simulink model "VCU_CS75_12_27_test_log"  (R2014a)
settings: Solver=FixedStepDiscrete  StartTime=0.0  StopTime=25  FixedStep=0.0005  RelTol=1e-3
undefined symbols (not defined in the file or in its folder): ecucoder_acal, ErrorSumMax1, ErrorSumMax2, ErrorSumMax3, I1, I2, I3, I_SW01_L, LaterlAngleCommand, LDW, Log_ErrorSumMax1, Log_ErrorSumMax2, Log_I1, Log_I2, Log_P1, Log_P2, Log_Takeover, P1, P2, P3, RemoteAcc, RemoteAcclPosition
libraries: simulink x927, ec5744lib x40
(part 4 of 31)

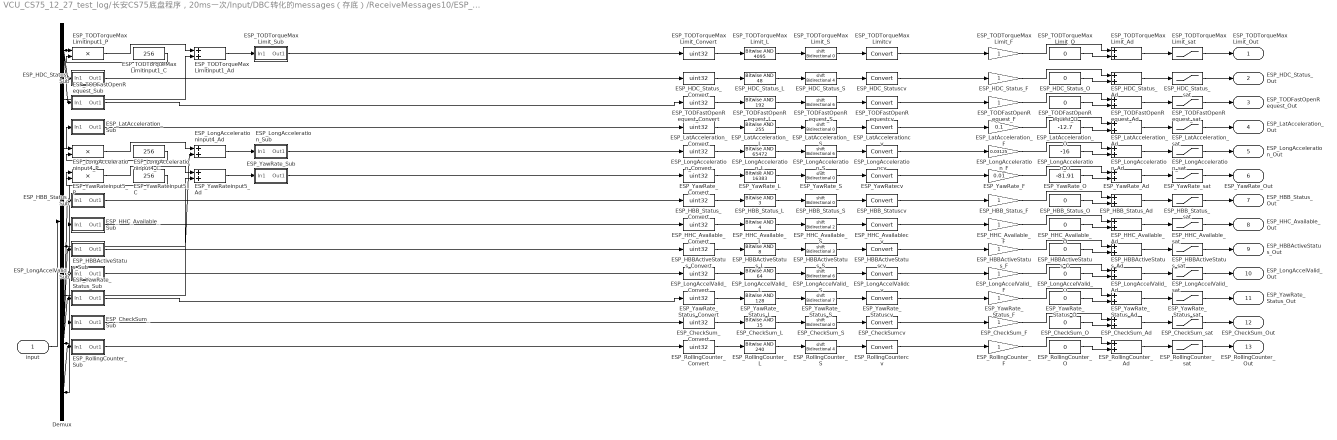
== system VCU_CS75_12_27_test_log/长安CS75底盘程序，20ms一次/Input/DBC转化的messages（存底）/ReceiveMessages10/ESP_287 ==
  input : Inport
  Demux : Demux  Outputs=8
  ESP_CheckSum_Ad : Sum
  ESP_CheckSum_Convert : DataTypeConversion  OutDataTypeStr=uint32
  ESP_CheckSum_F : Gain
  ESP_CheckSum_L : simulink/Logic and Bit Operations/Bitwise Operator  logicop=AND  UseBitMask=on  BitMask=15  BitMaskRealWorld=Stored Integer
  ESP_CheckSum_O : Constant  Value=0  OutDataTypeStr=single
  ESP_CheckSum_S : ArithShift
  ESP_CheckSum_Sub : Subsystem
  ESP_CheckSum_sat : Saturate  UpperLimit=15  LowerLimit=0
  ESP_CheckSumcv : DataTypeConversion
  ESP_HBBActiveStatus_Ad : Sum
  ESP_HBBActiveStatus_Convert : DataTypeConversion  OutDataTypeStr=uint32
  ESP_HBBActiveStatus_F : Gain
  ESP_HBBActiveStatus_L : simulink/Logic and Bit Operations/Bitwise Operator  logicop=AND  UseBitMask=on  BitMask=8  BitMaskRealWorld=Stored Integer
  ESP_HBBActiveStatus_O : Constant  Value=0  OutDataTypeStr=single
  ESP_HBBActiveStatus_S : ArithShift  BitShiftNumber=3
  ESP_HBBActiveStatus_Sub : Subsystem
  ESP_HBBActiveStatus_sat : Saturate  UpperLimit=1  LowerLimit=0
  ESP_HBBActiveStatuscv : DataTypeConversion
  ESP_HBB_Status_Ad : Sum
  ESP_HBB_Status_Convert : DataTypeConversion  OutDataTypeStr=uint32
  ESP_HBB_Status_F : Gain
  ESP_HBB_Status_L : simulink/Logic and Bit Operations/Bitwise Operator  logicop=AND  UseBitMask=on  BitMask=3  BitMaskRealWorld=Stored Integer
  ESP_HBB_Status_O : Constant  Value=0  OutDataTypeStr=single
  ESP_HBB_Status_S : ArithShift
  ESP_HBB_Status_Sub : Subsystem
  ESP_HBB_Status_sat : Saturate  UpperLimit=3  LowerLimit=0
  ESP_HBB_Statuscv : DataTypeConversion
  ESP_HDC_Status_Ad : Sum
  ESP_HDC_Status_Convert : DataTypeConversion  OutDataTypeStr=uint32
  ESP_HDC_Status_F : Gain
  ESP_HDC_Status_L : simulink/Logic and Bit Operations/Bitwise Operator  logicop=AND  UseBitMask=on  BitMask=48  BitMaskRealWorld=Stored Integer
  ESP_HDC_Status_O : Constant  Value=0  OutDataTypeStr=single
  ESP_HDC_Status_S : ArithShift  BitShiftNumber=4
  ESP_HDC_Status_Sub : Subsystem
  ESP_HDC_Status_sat : Saturate  UpperLimit=3  LowerLimit=0
  ESP_HDC_Statuscv : DataTypeConversion
  ESP_HHC_Available_Ad : Sum
  ESP_HHC_Available_Convert : DataTypeConversion  OutDataTypeStr=uint32
  ESP_HHC_Available_F : Gain
  ESP_HHC_Available_L : simulink/Logic and Bit Operations/Bitwise Operator  logicop=AND  UseBitMask=on  BitMask=4  BitMaskRealWorld=Stored Integer
  ESP_HHC_Available_O : Constant  Value=0  OutDataTypeStr=single
  ESP_HHC_Available_S : ArithShift  BitShiftNumber=2
  ESP_HHC_Available_Sub : Subsystem
  ESP_HHC_Available_sat : Saturate  UpperLimit=1  LowerLimit=0
  ESP_HHC_Availablecv : DataTypeConversion
  ESP_LatAcceleration_Ad : Sum
  ESP_LatAcceleration_Convert : DataTypeConversion  OutDataTypeStr=uint32
  ESP_LatAcceleration_F : Gain  Gain=0.1
  ESP_LatAcceleration_L : simulink/Logic and Bit Operations/Bitwise Operator  logicop=AND  UseBitMask=on  BitMask=255  BitMaskRealWorld=Stored Integer
  ESP_LatAcceleration_O : Constant  Value=-12.7  OutDataTypeStr=single
  ESP_LatAcceleration_S : ArithShift
  ESP_LatAcceleration_Sub : Subsystem
  ESP_LatAcceleration_sat : Saturate  UpperLimit=12.7  LowerLimit=-12.7
  ESP_LatAccelerationcv : DataTypeConversion
  ESP_LongAccelValid_Ad : Sum
  ESP_LongAccelValid_Convert : DataTypeConversion  OutDataTypeStr=uint32
  ESP_LongAccelValid_F : Gain
  ESP_LongAccelValid_L : simulink/Logic and Bit Operations/Bitwise Operator  logicop=AND  UseBitMask=on  BitMask=64  BitMaskRealWorld=Stored Integer
  ESP_LongAccelValid_O : Constant  Value=0  OutDataTypeStr=single
  ESP_LongAccelValid_S : ArithShift  BitShiftNumber=6
  ESP_LongAccelValid_Sub : Subsystem
  ESP_LongAccelValid_sat : Saturate  UpperLimit=1  LowerLimit=0
  ESP_LongAccelValidcv : DataTypeConversion
  ESP_LongAcceleration_Ad : Sum
  ESP_LongAcceleration_Convert : DataTypeConversion  OutDataTypeStr=uint32
  ESP_LongAcceleration_F : Gain  Gain=0.03125
  ESP_LongAcceleration_L : simulink/Logic and Bit Operations/Bitwise Operator  logicop=AND  UseBitMask=on  BitMask=65472  BitMaskRealWorld=Stored Integer
  ESP_LongAcceleration_O : Constant  Value=-16  OutDataTypeStr=single
  ESP_LongAcceleration_S : ArithShift  BitShiftNumber=6
  ESP_LongAcceleration_Sub : Subsystem
  ESP_LongAcceleration_sat : Saturate  UpperLimit=15.96875  LowerLimit=-16
  ESP_LongAccelerationcv : DataTypeConversion
  ESP_LongAccelerationinput4_Ad : Sum
  ESP_LongAccelerationinput4_C : Constant  Value=256
  ESP_LongAccelerationinput4_P : Product
  ESP_RollingCounter_Ad : Sum
  ESP_RollingCounter_Convert : DataTypeConversion  OutDataTypeStr=uint32
  ESP_RollingCounter_F : Gain
  ESP_RollingCounter_L : simulink/Logic and Bit Operations/Bitwise Operator  logicop=AND  UseBitMask=on  BitMask=240  BitMaskRealWorld=Stored Integer
  ESP_RollingCounter_O : Constant  Value=0  OutDataTypeStr=single
  ESP_RollingCounter_S : ArithShift  BitShiftNumber=4
  ESP_RollingCounter_Sub : Subsystem
  ESP_RollingCounter_sat : Saturate  UpperLimit=15  LowerLimit=0
  ESP_RollingCountercv : DataTypeConversion
  ESP_TODFastOpenRequest_Ad : Sum
  ESP_TODFastOpenRequest_Convert : DataTypeConversion  OutDataTypeStr=uint32
  ESP_TODFastOpenRequest_F : Gain
  ESP_TODFastOpenRequest_L : simulink/Logic and Bit Operations/Bitwise Operator  logicop=AND  UseBitMask=on  BitMask=192  BitMaskRealWorld=Stored Integer
  ESP_TODFastOpenRequest_O : Constant  Value=0  OutDataTypeStr=single
  ESP_TODFastOpenRequest_S : ArithShift  BitShiftNumber=6
  ESP_TODFastOpenRequest_Sub : Subsystem
  ESP_TODFastOpenRequest_sat : Saturate  UpperLimit=3  LowerLimit=0
  ESP_TODFastOpenRequestcv : DataTypeConversion
  ESP_TODTorqueMaxLimit_Ad : Sum
  ESP_TODTorqueMaxLimit_Convert : DataTypeConversion  OutDataTypeStr=uint32
  ESP_TODTorqueMaxLimit_F : Gain
  ESP_TODTorqueMaxLimit_L : simulink/Logic and Bit Operations/Bitwise Operator  logicop=AND  UseBitMask=on  BitMask=4095  BitMaskRealWorld=Stored Integer
  ESP_TODTorqueMaxLimit_O : Constant  Value=0  OutDataTypeStr=single
  ESP_TODTorqueMaxLimit_S : ArithShift
  ESP_TODTorqueMaxLimit_Sub : Subsystem
  ESP_TODTorqueMaxLimit_sat : Saturate  UpperLimit=4095  LowerLimit=0
  ESP_TODTorqueMaxLimitcv : DataTypeConversion
  ESP_TODTorqueMaxLimitinput1_Ad : Sum
  ESP_TODTorqueMaxLimitinput1_C : Constant  Value=256
  ESP_TODTorqueMaxLimitinput1_P : Product
  ESP_YawRate_Ad : Sum
  ESP_YawRate_Convert : DataTypeConversion  OutDataTypeStr=uint32
  ESP_YawRate_F : Gain  Gain=0.01
  ESP_YawRate_L : simulink/Logic and Bit Operations/Bitwise Operator  logicop=AND  UseBitMask=on  BitMask=16383  BitMaskRealWorld=Stored Integer
  ESP_YawRate_O : Constant  Value=-81.91  OutDataTypeStr=single
  ESP_YawRate_S : ArithShift
  ESP_YawRate_Status_Ad : Sum
  ESP_YawRate_Status_Convert : DataTypeConversion  OutDataTypeStr=uint32
  ESP_YawRate_Status_F : Gain
  ESP_YawRate_Status_L : simulink/Logic and Bit Operations/Bitwise Operator  logicop=AND  UseBitMask=on  BitMask=128  BitMaskRealWorld=Stored Integer
  ESP_YawRate_Status_O : Constant  Value=0  OutDataTypeStr=single
  ESP_YawRate_Status_S : ArithShift  BitShiftNumber=7
  ESP_YawRate_Status_Sub : Subsystem
  ESP_YawRate_Status_sat : Saturate  UpperLimit=1  LowerLimit=0
  ESP_YawRate_Statuscv : DataTypeConversion
  ESP_YawRate_Sub : Subsystem
  ESP_YawRate_sat : Saturate  UpperLimit=81.91  LowerLimit=-81.91
  ESP_YawRatecv : DataTypeConversion
  ESP_YawRateinput5_Ad : Sum
  ESP_YawRateinput5_C : Constant  Value=256
  ESP_YawRateinput5_P : Product
  ESP_TODTorqueMaxLimit_Out : Outport
  ESP_HDC_Status_Out : Outport  Port=2
  ESP_TODFastOpenRequest_Out : Outport  Port=3
  ESP_LatAcceleration_Out : Outport  Port=4
  ESP_LongAcceleration_Out : Outport  Port=5
  ESP_YawRate_Out : Outport  Port=6
  ESP_HBB_Status_Out : Outport  Port=7
  ESP_HHC_Available_Out : Outport  Port=8
  ESP_HBBActiveStatus_Out : Outport  Port=9
  ESP_LongAccelValid_Out : Outport  Port=10
  ESP_YawRate_Status_Out : Outport  Port=11
  ESP_CheckSum_Out : Outport  Port=12
  ESP_RollingCounter_Out : Outport  Port=13
  wires:
  input/1 -> Demux/1
  ESP_RollingCountercv/1 -> ESP_RollingCounter_F/1
  ESP_RollingCounter_S/1 -> ESP_RollingCountercv/1
  ESP_RollingCounter_L/1 -> ESP_RollingCounter_S/1
  ESP_RollingCounter_Convert/1 -> ESP_RollingCounter_L/1
  ESP_RollingCounter_Sub/1(Out1) -> ESP_RollingCounter_Convert/1
  ESP_RollingCounter_sat/1 -> ESP_RollingCounter_Out/1
  ESP_RollingCounter_Ad/1 -> ESP_RollingCounter_sat/1
  ESP_RollingCounter_O/1 -> ESP_RollingCounter_Ad/2
  ESP_RollingCounter_F/1 -> ESP_RollingCounter_Ad/1
  ESP_CheckSumcv/1 -> ESP_CheckSum_F/1
  ESP_CheckSum_S/1 -> ESP_CheckSumcv/1
  ESP_CheckSum_L/1 -> ESP_CheckSum_S/1
  ESP_CheckSum_Convert/1 -> ESP_CheckSum_L/1
  ESP_CheckSum_Sub/1(Out1) -> ESP_CheckSum_Convert/1
  Demux/8 -> ESP_RollingCounter_Sub/1(In1), ESP_CheckSum_Sub/1(In1)
  ESP_CheckSum_sat/1 -> ESP_CheckSum_Out/1
  ESP_CheckSum_Ad/1 -> ESP_CheckSum_sat/1
  ESP_CheckSum_O/1 -> ESP_CheckSum_Ad/2
  ESP_CheckSum_F/1 -> ESP_CheckSum_Ad/1
  ESP_YawRate_Statuscv/1 -> ESP_YawRate_Status_F/1
  ESP_YawRate_Status_S/1 -> ESP_YawRate_Statuscv/1
  ESP_YawRate_Status_L/1 -> ESP_YawRate_Status_S/1
  ESP_YawRate_Status_Convert/1 -> ESP_YawRate_Status_L/1
  ESP_YawRate_Status_Sub/1(Out1) -> ESP_YawRate_Status_Convert/1
  ESP_YawRate_Status_sat/1 -> ESP_YawRate_Status_Out/1
  ESP_YawRate_Status_Ad/1 -> ESP_YawRate_Status_sat/1
  ESP_YawRate_Status_O/1 -> ESP_YawRate_Status_Ad/2
  ESP_YawRate_Status_F/1 -> ESP_YawRate_Status_Ad/1
  ESP_LongAccelValidcv/1 -> ESP_LongAccelValid_F/1
  ESP_LongAccelValid_S/1 -> ESP_LongAccelValidcv/1
  ESP_LongAccelValid_L/1 -> ESP_LongAccelValid_S/1
  ESP_LongAccelValid_Convert/1 -> ESP_LongAccelValid_L/1
  ESP_LongAccelValid_Sub/1(Out1) -> ESP_LongAccelValid_Convert/1
  ESP_LongAccelValid_sat/1 -> ESP_LongAccelValid_Out/1
  ESP_LongAccelValid_Ad/1 -> ESP_LongAccelValid_sat/1
  ESP_LongAccelValid_O/1 -> ESP_LongAccelValid_Ad/2
  ESP_LongAccelValid_F/1 -> ESP_LongAccelValid_Ad/1
  ESP_HBBActiveStatuscv/1 -> ESP_HBBActiveStatus_F/1
  ESP_HBBActiveStatus_S/1 -> ESP_HBBActiveStatuscv/1
  ESP_HBBActiveStatus_L/1 -> ESP_HBBActiveStatus_S/1
  ESP_HBBActiveStatus_Convert/1 -> ESP_HBBActiveStatus_L/1
  ESP_HBBActiveStatus_Sub/1(Out1) -> ESP_HBBActiveStatus_Convert/1
  ESP_HBBActiveStatus_sat/1 -> ESP_HBBActiveStatus_Out/1
  ESP_HBBActiveStatus_Ad/1 -> ESP_HBBActiveStatus_sat/1
  ESP_HBBActiveStatus_O/1 -> ESP_HBBActiveStatus_Ad/2
  ESP_HBBActiveStatus_F/1 -> ESP_HBBActiveStatus_Ad/1
  ESP_HHC_Availablecv/1 -> ESP_HHC_Available_F/1
  ESP_HHC_Available_S/1 -> ESP_HHC_Availablecv/1
  ESP_HHC_Available_L/1 -> ESP_HHC_Available_S/1
  ESP_HHC_Available_Convert/1 -> ESP_HHC_Available_L/1
  ESP_HHC_Available_Sub/1(Out1) -> ESP_HHC_Available_Convert/1
  ESP_HHC_Available_sat/1 -> ESP_HHC_Available_Out/1
  ESP_HHC_Available_Ad/1 -> ESP_HHC_Available_sat/1
  ESP_HHC_Available_O/1 -> ESP_HHC_Available_Ad/2
  ESP_HHC_Available_F/1 -> ESP_HHC_Available_Ad/1
  ESP_HBB_Statuscv/1 -> ESP_HBB_Status_F/1
  ESP_HBB_Status_S/1 -> ESP_HBB_Statuscv/1
  ESP_HBB_Status_L/1 -> ESP_HBB_Status_S/1
  ESP_HBB_Status_Convert/1 -> ESP_HBB_Status_L/1
  ESP_HBB_Status_Sub/1(Out1) -> ESP_HBB_Status_Convert/1
  Demux/7 -> ESP_YawRate_Status_Sub/1(In1), ESP_LongAccelValid_Sub/1(In1), ESP_HBBActiveStatus_Sub/1(In1), ESP_HHC_Available_Sub/1(In1), ESP_HBB_Status_Sub/1(In1)
  ESP_HBB_Status_sat/1 -> ESP_HBB_Status_Out/1
  ESP_HBB_Status_Ad/1 -> ESP_HBB_Status_sat/1
  ESP_HBB_Status_O/1 -> ESP_HBB_Status_Ad/2
  ESP_HBB_Status_F/1 -> ESP_HBB_Status_Ad/1
  ESP_YawRatecv/1 -> ESP_YawRate_F/1
  ESP_YawRate_S/1 -> ESP_YawRatecv/1
  ESP_YawRate_L/1 -> ESP_YawRate_S/1
  ESP_YawRate_Convert/1 -> ESP_YawRate_L/1
  ESP_YawRate_Sub/1(Out1) -> ESP_YawRate_Convert/1
  ESP_YawRateinput5_Ad/1 -> ESP_YawRate_Sub/1(In1)
  Demux/6 -> ESP_YawRateinput5_Ad/2
  ESP_YawRateinput5_P/1 -> ESP_YawRateinput5_Ad/1
  ESP_YawRateinput5_C/1 -> ESP_YawRateinput5_P/2
  ESP_YawRate_sat/1 -> ESP_YawRate_Out/1
  ESP_YawRate_Ad/1 -> ESP_YawRate_sat/1
  ESP_YawRate_O/1 -> ESP_YawRate_Ad/2
  ESP_YawRate_F/1 -> ESP_YawRate_Ad/1
  ESP_LongAccelerationcv/1 -> ESP_LongAcceleration_F/1
  ESP_LongAcceleration_S/1 -> ESP_LongAccelerationcv/1
  ESP_LongAcceleration_L/1 -> ESP_LongAcceleration_S/1
  ESP_LongAcceleration_Convert/1 -> ESP_LongAcceleration_L/1
  ESP_LongAcceleration_Sub/1(Out1) -> ESP_LongAcceleration_Convert/1
  ESP_LongAccelerationinput4_Ad/1 -> ESP_LongAcceleration_Sub/1(In1)
  Demux/5 -> ESP_YawRateinput5_P/1, ESP_LongAccelerationinput4_Ad/2
  ESP_LongAccelerationinput4_P/1 -> ESP_LongAccelerationinput4_Ad/1
  ESP_LongAccelerationinput4_C/1 -> ESP_LongAccelerationinput4_P/2
  Demux/4 -> ESP_LongAccelerationinput4_P/1
  ESP_LongAcceleration_sat/1 -> ESP_LongAcceleration_Out/1
  ESP_LongAcceleration_Ad/1 -> ESP_LongAcceleration_sat/1
  ESP_LongAcceleration_O/1 -> ESP_LongAcceleration_Ad/2
  ESP_LongAcceleration_F/1 -> ESP_LongAcceleration_Ad/1
  ESP_LatAccelerationcv/1 -> ESP_LatAcceleration_F/1
  ESP_LatAcceleration_S/1 -> ESP_LatAccelerationcv/1
  ESP_LatAcceleration_L/1 -> ESP_LatAcceleration_S/1
  ESP_LatAcceleration_Convert/1 -> ESP_LatAcceleration_L/1
  ESP_LatAcceleration_Sub/1(Out1) -> ESP_LatAcceleration_Convert/1
  Demux/3 -> ESP_LatAcceleration_Sub/1(In1)
  ESP_LatAcceleration_sat/1 -> ESP_LatAcceleration_Out/1
  ESP_LatAcceleration_Ad/1 -> ESP_LatAcceleration_sat/1
  ESP_LatAcceleration_O/1 -> ESP_LatAcceleration_Ad/2
  ESP_LatAcceleration_F/1 -> ESP_LatAcceleration_Ad/1
  ESP_TODFastOpenRequestcv/1 -> ESP_TODFastOpenRequest_F/1
  ESP_TODFastOpenRequest_S/1 -> ESP_TODFastOpenRequestcv/1
  ESP_TODFastOpenRequest_L/1 -> ESP_TODFastOpenRequest_S/1
  ESP_TODFastOpenRequest_Convert/1 -> ESP_TODFastOpenRequest_L/1
  ESP_TODFastOpenRequest_Sub/1(Out1) -> ESP_TODFastOpenRequest_Convert/1
  ESP_TODFastOpenRequest_sat/1 -> ESP_TODFastOpenRequest_Out/1
  ESP_TODFastOpenRequest_Ad/1 -> ESP_TODFastOpenRequest_sat/1
  ESP_TODFastOpenRequest_O/1 -> ESP_TODFastOpenRequest_Ad/2
  ESP_TODFastOpenRequest_F/1 -> ESP_TODFastOpenRequest_Ad/1
  ESP_HDC_Statuscv/1 -> ESP_HDC_Status_F/1
  ESP_HDC_Status_S/1 -> ESP_HDC_Statuscv/1
  ESP_HDC_Status_L/1 -> ESP_HDC_Status_S/1
  ESP_HDC_Status_Convert/1 -> ESP_HDC_Status_L/1
  ESP_HDC_Status_Sub/1(Out1) -> ESP_HDC_Status_Convert/1
  ESP_HDC_Status_sat/1 -> ESP_HDC_Status_Out/1
  ESP_HDC_Status_Ad/1 -> ESP_HDC_Status_sat/1
  ESP_HDC_Status_O/1 -> ESP_HDC_Status_Ad/2
  ESP_HDC_Status_F/1 -> ESP_HDC_Status_Ad/1
  ESP_TODTorqueMaxLimitcv/1 -> ESP_TODTorqueMaxLimit_F/1
  ESP_TODTorqueMaxLimit_S/1 -> ESP_TODTorqueMaxLimitcv/1
  ESP_TODTorqueMaxLimit_L/1 -> ESP_TODTorqueMaxLimit_S/1
  ESP_TODTorqueMaxLimit_Convert/1 -> ESP_TODTorqueMaxLimit_L/1
  ESP_TODTorqueMaxLimit_Sub/1(Out1) -> ESP_TODTorqueMaxLimit_Convert/1
  ESP_TODTorqueMaxLimitinput1_Ad/1 -> ESP_TODTorqueMaxLimit_Sub/1(In1)
  Demux/2 -> ESP_TODTorqueMaxLimitinput1_Ad/2
  ESP_TODTorqueMaxLimitinput1_P/1 -> ESP_TODTorqueMaxLimitinput1_Ad/1
  ESP_TODTorqueMaxLimitinput1_C/1 -> ESP_TODTorqueMaxLimitinput1_P/2
  Demux/1 -> ESP_TODFastOpenRequest_Sub/1(In1), ESP_HDC_Status_Sub/1(In1), ESP_TODTorqueMaxLimitinput1_P/1
  ESP_TODTorqueMaxLimit_sat/1 -> ESP_TODTorqueMaxLimit_Out/1
  ESP_TODTorqueMaxLimit_Ad/1 -> ESP_TODTorqueMaxLimit_sat/1
  ESP_TODTorqueMaxLimit_O/1 -> ESP_TODTorqueMaxLimit_Ad/2
  ESP_TODTorqueMaxLimit_F/1 -> ESP_TODTorqueMaxLimit_Ad/1

== system VCU_CS75_12_27_test_log/长安CS75底盘程序，20ms一次/Input/DBC转化的messages（存底）/ReceiveMessages11/HU_AEBSetting_551 ==
  input : Inport
  Demux : Demux  Outputs=8
  HU_AEBOnOffSetting_Ad : Sum
  HU_AEBOnOffSetting_Convert : DataTypeConversion  OutDataTypeStr=uint32
  HU_AEBOnOffSetting_F : Gain
  HU_AEBOnOffSetting_L : simulink/Logic and Bit Operations/Bitwise Operator  logicop=AND  UseBitMask=on  BitMask=8  BitMaskRealWorld=Stored Integer
  HU_AEBOnOffSetting_O : Constant  Value=0  OutDataTypeStr=single
  HU_AEBOnOffSetting_S : ArithShift  BitShiftNumber=3
  HU_AEBOnOffSetting_Sub : Subsystem
  HU_AEBOnOffSetting_sat : Saturate  UpperLimit=1  LowerLimit=0
  HU_AEBOnOffSettingcv : DataTypeConversion
  HU_FCWSetting_Ad : Sum
  HU_FCWSetting_Convert : DataTypeConversion  OutDataTypeStr=uint32
  HU_FCWSetting_F : Gain
  HU_FCWSetting_L : simulink/Logic and Bit Operations/Bitwise Operator  logicop=AND  UseBitMask=on  BitMask=24  BitMaskRealWorld=Stored Integer
  HU_FCWSetting_O : Constant  Value=0  OutDataTypeStr=single
  HU_FCWSetting_S : ArithShift  BitShiftNumber=3
  HU_FCWSetting_Sub : Subsystem
  HU_FCWSetting_sat : Saturate  UpperLimit=0  LowerLimit=0
  HU_FCWSettingcv : DataTypeConversion
  HU_LCASetting_Ad : Sum
  HU_LCASetting_Convert : DataTypeConversion  OutDataTypeStr=uint32
  HU_LCASetting_F : Gain
  HU_LCASetting_L : simulink/Logic and Bit Operations/Bitwise Operator  logicop=AND  UseBitMask=on  BitMask=3  BitMaskRealWorld=Stored Integer
  HU_LCASetting_O : Constant  Value=0  OutDataTypeStr=single
  HU_LCASetting_S : ArithShift
  HU_LCASetting_Sub : Subsystem
  HU_LCASetting_sat : Saturate  UpperLimit=0  LowerLimit=0
  HU_LCASettingcv : DataTypeConversion
  HU_AEBOnOffSetting_Out : Outport
  HU_LCASetting_Out : Outport  Port=2
  HU_FCWSetting_Out : Outport  Port=3
  wires:
  input/1 -> Demux/1
  HU_FCWSettingcv/1 -> HU_FCWSetting_F/1
  HU_FCWSetting_S/1 -> HU_FCWSettingcv/1
  HU_FCWSetting_L/1 -> HU_FCWSetting_S/1
  HU_FCWSetting_Convert/1 -> HU_FCWSetting_L/1
  HU_FCWSetting_Sub/1(Out1) -> HU_FCWSetting_Convert/1
  HU_FCWSetting_sat/1 -> HU_FCWSetting_Out/1
  HU_FCWSetting_Ad/1 -> HU_FCWSetting_sat/1
  HU_FCWSetting_O/1 -> HU_FCWSetting_Ad/2
  HU_FCWSetting_F/1 -> HU_FCWSetting_Ad/1
  HU_LCASettingcv/1 -> HU_LCASetting_F/1
  HU_LCASetting_S/1 -> HU_LCASettingcv/1
  HU_LCASetting_L/1 -> HU_LCASetting_S/1
  HU_LCASetting_Convert/1 -> HU_LCASetting_L/1
  HU_LCASetting_Sub/1(Out1) -> HU_LCASetting_Convert/1
  Demux/5 -> HU_FCWSetting_Sub/1(In1), HU_LCASetting_Sub/1(In1)
  HU_LCASetting_sat/1 -> HU_LCASetting_Out/1
  HU_LCASetting_Ad/1 -> HU_LCASetting_sat/1
  HU_LCASetting_O/1 -> HU_LCASetting_Ad/2
  HU_LCASetting_F/1 -> HU_LCASetting_Ad/1
  HU_AEBOnOffSettingcv/1 -> HU_AEBOnOffSetting_F/1
  HU_AEBOnOffSetting_S/1 -> HU_AEBOnOffSettingcv/1
  HU_AEBOnOffSetting_L/1 -> HU_AEBOnOffSetting_S/1
  HU_AEBOnOffSetting_Convert/1 -> HU_AEBOnOffSetting_L/1
  HU_AEBOnOffSetting_Sub/1(Out1) -> HU_AEBOnOffSetting_Convert/1
  Demux/1 -> HU_AEBOnOffSetting_Sub/1(In1)
  HU_AEBOnOffSetting_sat/1 -> HU_AEBOnOffSetting_Out/1
  HU_AEBOnOffSetting_Ad/1 -> HU_AEBOnOffSetting_sat/1
  HU_AEBOnOffSetting_O/1 -> HU_AEBOnOffSetting_Ad/2
  HU_AEBOnOffSetting_F/1 -> HU_AEBOnOffSetting_Ad/1

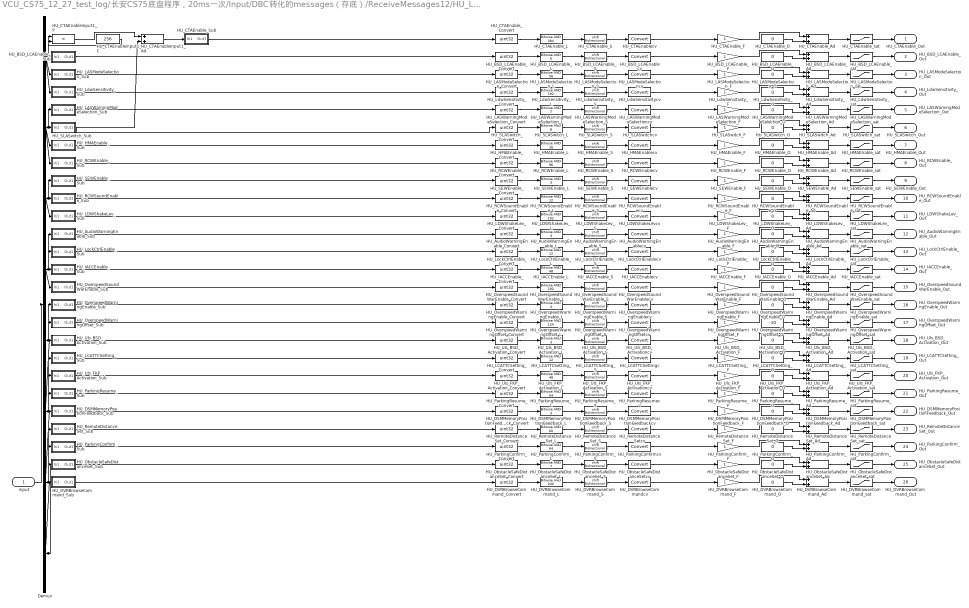
== system VCU_CS75_12_27_test_log/长安CS75底盘程序，20ms一次/Input/DBC转化的messages（存底）/ReceiveMessages12/HU_LASSetting_0x541 ==
  input : Inport
  Demux : Demux  Outputs=8
  HU_AudioWarningEnable_Ad : Sum
  HU_AudioWarningEnable_Convert : DataTypeConversion  OutDataTypeStr=uint32
  HU_AudioWarningEnable_F : Gain
  HU_AudioWarningEnable_L : simulink/Logic and Bit Operations/Bitwise Operator  logicop=AND  UseBitMask=on  BitMask=3  BitMaskRealWorld=Stored Integer
  HU_AudioWarningEnable_O : Constant  Value=0  OutDataTypeStr=single
  HU_AudioWarningEnable_S : ArithShift
  HU_AudioWarningEnable_Sub : Subsystem
  HU_AudioWarningEnable_sat : Saturate  UpperLimit=3  LowerLimit=0
  HU_AudioWarningEnablecv : DataTypeConversion
  HU_BSD_LCAEnable_Ad : Sum
  HU_BSD_LCAEnable_Convert : DataTypeConversion  OutDataTypeStr=uint32
  HU_BSD_LCAEnable_F : Gain
  HU_BSD_LCAEnable_L : simulink/Logic and Bit Operations/Bitwise Operator  logicop=AND  UseBitMask=on  BitMask=6  BitMaskRealWorld=Stored Integer
  HU_BSD_LCAEnable_O : Constant  Value=0  OutDataTypeStr=single
  HU_BSD_LCAEnable_S : ArithShift  BitShiftNumber=1
  HU_BSD_LCAEnable_Sub : Subsystem
  HU_BSD_LCAEnable_sat : Saturate  UpperLimit=3  LowerLimit=0
  HU_BSD_LCAEnablecv : DataTypeConversion
  HU_CTAEnable_Ad : Sum
  HU_CTAEnable_Convert : DataTypeConversion  OutDataTypeStr=uint32
  HU_CTAEnable_F : Gain
  HU_CTAEnable_L : simulink/Logic and Bit Operations/Bitwise Operator  logicop=AND  UseBitMask=on  BitMask=384  BitMaskRealWorld=Stored Integer
  HU_CTAEnable_O : Constant  Value=0  OutDataTypeStr=single
  HU_CTAEnable_S : ArithShift  BitShiftNumber=7
  HU_CTAEnable_Sub : Subsystem
  HU_CTAEnable_sat : Saturate  UpperLimit=3  LowerLimit=0
  HU_CTAEnablecv : DataTypeConversion
  HU_CTAEnableinput1_Ad : Sum
  HU_CTAEnableinput1_C : Constant  Value=256
  HU_CTAEnableinput1_P : Product
  HU_DSMMemoryPositionFeedback_Ad : Sum
  HU_DSMMemoryPositionFeedback_Convert : DataTypeConversion  OutDataTypeStr=uint32
  HU_DSMMemoryPositionFeedback_F : Gain
  HU_DSMMemoryPositionFeedback_L : simulink/Logic and Bit Operations/Bitwise Operator  logicop=AND  UseBitMask=on  BitMask=3  BitMaskRealWorld=Stored Integer
  HU_DSMMemoryPositionFeedback_O : Constant  Value=0  OutDataTypeStr=single
  HU_DSMMemoryPositionFeedback_S : ArithShift
  HU_DSMMemoryPositionFeedback_Sub : Subsystem
  HU_DSMMemoryPositionFeedback_sat : Saturate  UpperLimit=3  LowerLimit=0
  HU_DSMMemoryPositionFeedbackcv : DataTypeConversion
  HU_DVRBrowseCommand_Ad : Sum
  HU_DVRBrowseCommand_Convert : DataTypeConversion  OutDataTypeStr=uint32
  HU_DVRBrowseCommand_F : Gain
  HU_DVRBrowseCommand_L : simulink/Logic and Bit Operations/Bitwise Operator  logicop=AND  UseBitMask=on  BitMask=240  BitMaskRealWorld=Stored Integer
  HU_DVRBrowseCommand_O : Constant  Value=0  OutDataTypeStr=single
  HU_DVRBrowseCommand_S : ArithShift  BitShiftNumber=4
  HU_DVRBrowseCommand_Sub : Subsystem
  HU_DVRBrowseCommand_sat : Saturate  UpperLimit=15  LowerLimit=0
  HU_DVRBrowseCommandcv : DataTypeConversion
  HU_HMAEnable_Ad : Sum
  HU_HMAEnable_Convert : DataTypeConversion  OutDataTypeStr=uint32
  HU_HMAEnable_F : Gain
  HU_HMAEnable_L : simulink/Logic and Bit Operations/Bitwise Operator  logicop=AND  UseBitMask=on  BitMask=16  BitMaskRealWorld=Stored Integer
  HU_HMAEnable_O : Constant  Value=0  OutDataTypeStr=single
  HU_HMAEnable_S : ArithShift  BitShiftNumber=4
  HU_HMAEnable_Sub : Subsystem
  HU_HMAEnable_sat : Saturate  UpperLimit=1  LowerLimit=0
  HU_HMAEnablecv : DataTypeConversion
  HU_IACCEnable_Ad : Sum
  HU_IACCEnable_Convert : DataTypeConversion  OutDataTypeStr=uint32
  HU_IACCEnable_F : Gain
  HU_IACCEnable_L : simulink/Logic and Bit Operations/Bitwise Operator  logicop=AND  UseBitMask=on  BitMask=48  BitMaskRealWorld=Stored Integer
  HU_IACCEnable_O : Constant  Value=0  OutDataTypeStr=single
  HU_IACCEnable_S : ArithShift  BitShiftNumber=4
  HU_IACCEnable_Sub : Subsystem
  HU_IACCEnable_sat : Saturate  UpperLimit=3  LowerLimit=0
  HU_IACCEnablecv : DataTypeConversion
  HU_LASModeSelection_Ad : Sum
  HU_LASModeSelection_Convert : DataTypeConversion  OutDataTypeStr=uint32
  HU_LASModeSelection_F : Gain
  HU_LASModeSelection_L : simulink/Logic and Bit Operations/Bitwise Operator  logicop=AND  UseBitMask=on  BitMask=56  BitMaskRealWorld=Stored Integer
  HU_LASModeSelection_O : Constant  Value=0  OutDataTypeStr=single
  HU_LASModeSelection_S : ArithShift  BitShiftNumber=3
  HU_LASModeSelection_Sub : Subsystem
  HU_LASModeSelection_sat : Saturate  UpperLimit=7  LowerLimit=0
  HU_LASModeSelectioncv : DataTypeConversion
  HU_LASWarningModeSelection_Ad : Sum
  HU_LASWarningModeSelection_Convert : DataTypeConversion  OutDataTypeStr=uint32
  HU_LASWarningModeSelection_F : Gain
  HU_LASWarningModeSelection_L : simulink/Logic and Bit Operations/Bitwise Operator  logicop=AND  UseBitMask=on  BitMask=7  BitMaskRealWorld=Stored Integer
  HU_LASWarningModeSelection_O : Constant  Value=0  OutDataTypeStr=single
  HU_LASWarningModeSelection_S : ArithShift
  HU_LASWarningModeSelection_Sub : Subsystem
  HU_LASWarningModeSelection_sat : Saturate  UpperLimit=7  LowerLimit=0
  HU_LASWarningModeSelectioncv : DataTypeConversion
  HU_LCATTCSetting_Ad : Sum
  HU_LCATTCSetting_Convert : DataTypeConversion  OutDataTypeStr=uint32
  HU_LCATTCSetting_F : Gain
  HU_LCATTCSetting_L : simulink/Logic and Bit Operations/Bitwise Operator  logicop=AND  UseBitMask=on  BitMask=12  BitMaskRealWorld=Stored Integer
  HU_LCATTCSetting_O : Constant  Value=0  OutDataTypeStr=single
  HU_LCATTCSetting_S : ArithShift  BitShiftNumber=2
  HU_LCATTCSetting_Sub : Subsystem
  HU_LCATTCSetting_sat : Saturate  UpperLimit=3  LowerLimit=0
  HU_LCATTCSettingcv : DataTypeConversion
  HU_LDWShakeLev_Ad : Sum
  HU_LDWShakeLev_Convert : DataTypeConversion  OutDataTypeStr=uint32
  HU_LDWShakeLev_F : Gain
  HU_LDWShakeLev_L : simulink/Logic and Bit Operations/Bitwise Operator  logicop=AND  UseBitMask=on  BitMask=192  BitMaskRealWorld=Stored Integer
  HU_LDWShakeLev_O : Constant  Value=0  OutDataTypeStr=single
  HU_LDWShakeLev_S : ArithShift  BitShiftNumber=6
  HU_LDWShakeLev_Sub : Subsystem
  HU_LDWShakeLev_sat : Saturate  UpperLimit=3  LowerLimit=0
  HU_LDWShakeLevcv : DataTypeConversion
  HU_LdwSensitivity_Ad : Sum
  HU_LdwSensitivity_Convert : DataTypeConversion  OutDataTypeStr=uint32
  HU_LdwSensitivity_F : Gain
  HU_LdwSensitivity_L : simulink/Logic and Bit Operations/Bitwise Operator  logicop=AND  UseBitMask=on  BitMask=192  BitMaskRealWorld=Stored Integer
  HU_LdwSensitivity_O : Constant  Value=0  OutDataTypeStr=single
  HU_LdwSensitivity_S : ArithShift  BitShiftNumber=6
  HU_LdwSensitivity_Sub : Subsystem
  HU_LdwSensitivity_sat : Saturate  UpperLimit=3  LowerLimit=0
  HU_LdwSensitivitycv : DataTypeConversion
  HU_LockCtrlEnable_Ad : Sum
  HU_LockCtrlEnable_Convert : DataTypeConversion  OutDataTypeStr=uint32
  HU_LockCtrlEnable_F : Gain
  HU_LockCtrlEnable_L : simulink/Logic and Bit Operations/Bitwise Operator  logicop=AND  UseBitMask=on  BitMask=12  BitMaskRealWorld=Stored Integer
  HU_LockCtrlEnable_O : Constant  Value=0  OutDataTypeStr=single
  HU_LockCtrlEnable_S : ArithShift  BitShiftNumber=2
  HU_LockCtrlEnable_Sub : Subsystem
  HU_LockCtrlEnable_sat : Saturate  UpperLimit=3  LowerLimit=0
  HU_LockCtrlEnablecv : DataTypeConversion
  HU_ObstacleSafeDistanceSet_Ad : Sum
  HU_ObstacleSafeDistanceSet_Convert : DataTypeConversion  OutDataTypeStr=uint32
  HU_ObstacleSafeDistanceSet_F : Gain
  HU_ObstacleSafeDistanceSet_L : simulink/Logic and Bit Operations/Bitwise Operator  logicop=AND  UseBitMask=on  BitMask=7  BitMaskRealWorld=Stored Integer
  HU_ObstacleSafeDistanceSet_O : Constant  Value=0  OutDataTypeStr=single
  HU_ObstacleSafeDistanceSet_S : ArithShift
  HU_ObstacleSafeDistanceSet_Sub : Subsystem
  HU_ObstacleSafeDistanceSet_sat : Saturate  UpperLimit=7  LowerLimit=0
  HU_ObstacleSafeDistanceSetcv : DataTypeConversion
  HU_OverspeedSoundWarEnable_Ad : Sum
  HU_OverspeedSoundWarEnable_Convert : DataTypeConversion  OutDataTypeStr=uint32
  HU_OverspeedSoundWarEnable_F : Gain
  HU_OverspeedSoundWarEnable_L : simulink/Logic and Bit Operations/Bitwise Operator  logicop=AND  UseBitMask=on  BitMask=192  BitMaskRealWorld=Stored Integer
  HU_OverspeedSoundWarEnable_O : Constant  Value=0  OutDataTypeStr=single
  HU_OverspeedSoundWarEnable_S : ArithShift  BitShiftNumber=6
  HU_OverspeedSoundWarEnable_Sub : Subsystem
  HU_OverspeedSoundWarEnable_sat : Saturate  UpperLimit=3  LowerLimit=0
  HU_OverspeedSoundWarEnablecv : DataTypeConversion
  HU_OverspeedWarningEnable_Ad : Sum
  HU_OverspeedWarningEnable_Convert : DataTypeConversion  OutDataTypeStr=uint32
  HU_OverspeedWarningEnable_F : Gain
  HU_OverspeedWarningEnable_L : simulink/Logic and Bit Operations/Bitwise Operator  logicop=AND  UseBitMask=on  BitMask=3  BitMaskRealWorld=Stored Integer
  HU_OverspeedWarningEnable_O : Constant  Value=0  OutDataTypeStr=single
  HU_OverspeedWarningEnable_S : ArithShift
  HU_OverspeedWarningEnable_Sub : Subsystem
  HU_OverspeedWarningEnable_sat : Saturate  UpperLimit=3  LowerLimit=0
  HU_OverspeedWarningEnablecv : DataTypeConversion
  HU_OverspeedWarningOffset_Ad : Sum
  HU_OverspeedWarningOffset_Convert : DataTypeConversion  OutDataTypeStr=uint32
  HU_OverspeedWarningOffset_F : Gain
  HU_OverspeedWarningOffset_L : simulink/Logic and Bit Operations/Bitwise Operator  logicop=AND  UseBitMask=on  BitMask=124  BitMaskRealWorld=Stored Integer
  HU_OverspeedWarningOffset_O : Constant  Value=-10  OutDataTypeStr=single
  HU_OverspeedWarningOffset_S : ArithShift  BitShiftNumber=2
  HU_OverspeedWarningOffset_Sub : Subsystem
  HU_OverspeedWarningOffset_sat : Saturate  UpperLimit=10  LowerLimit=-10
  HU_OverspeedWarningOffsetcv : DataTypeConversion
  HU_ParkingConfirm_Ad : Sum
  HU_ParkingConfirm_Convert : DataTypeConversion  OutDataTypeStr=uint32
  HU_ParkingConfirm_F : Gain
  HU_ParkingConfirm_L : simulink/Logic and Bit Operations/Bitwise Operator  logicop=AND  UseBitMask=on  BitMask=64  BitMaskRealWorld=Stored Integer
  HU_ParkingConfirm_O : Constant  Value=0  OutDataTypeStr=single
  HU_ParkingConfirm_S : ArithShift  BitShiftNumber=6
  HU_ParkingConfirm_Sub : Subsystem
  HU_ParkingConfirm_sat : Saturate  UpperLimit=1  LowerLimit=0
  HU_ParkingConfirmcv : DataTypeConversion
  HU_ParkingResume_Ad : Sum
  HU_ParkingResume_Convert : DataTypeConversion  OutDataTypeStr=uint32
  HU_ParkingResume_F : Gain
  HU_ParkingResume_L : simulink/Logic and Bit Operations/Bitwise Operator  logicop=AND  UseBitMask=on  BitMask=64  BitMaskRealWorld=Stored Integer
  HU_ParkingResume_O : Constant  Value=0  OutDataTypeStr=single
  HU_ParkingResume_S : ArithShift  BitShiftNumber=6
  HU_ParkingResume_Sub : Subsystem
  HU_ParkingResume_sat : Saturate  UpperLimit=1  LowerLimit=0
  HU_ParkingResumecv : DataTypeConversion
  HU_RCWEnable_Ad : Sum
  HU_RCWEnable_Convert : DataTypeConversion  OutDataTypeStr=uint32
  HU_RCWEnable_F : Gain
  HU_RCWEnable_L : simulink/Logic and Bit Operations/Bitwise Operator  logicop=AND  UseBitMask=on  BitMask=96  BitMaskRealWorld=Stored Integer
  HU_RCWEnable_O : Constant  Value=0  OutDataTypeStr=single
  HU_RCWEnable_S : ArithShift  BitShiftNumber=5
  HU_RCWEnable_Sub : Subsystem
  HU_RCWEnable_sat : Saturate  UpperLimit=3  LowerLimit=0
  HU_RCWEnablecv : DataTypeConversion
  HU_RCWSoundEnable_Ad : Sum
  HU_RCWSoundEnable_Convert : DataTypeConversion  OutDataTypeStr=uint32
  HU_RCWSoundEnable_F : Gain
  HU_RCWSoundEnable_L : simulink/Logic and Bit Operations/Bitwise Operator  logicop=AND  UseBitMask=on  BitMask=12  BitMaskRealWorld=Stored Integer
  HU_RCWSoundEnable_O : Constant  Value=0  OutDataTypeStr=single
  HU_RCWSoundEnable_S : ArithShift  BitShiftNumber=2
  HU_RCWSoundEnable_Sub : Subsystem
  HU_RCWSoundEnable_sat : Saturate  UpperLimit=3  LowerLimit=0
  HU_RCWSoundEnablecv : DataTypeConversion
  HU_RemoteDistanceSet_Ad : Sum
  HU_RemoteDistanceSet_Convert : DataTypeConversion  OutDataTypeStr=uint32
  HU_RemoteDistanceSet_F : Gain
  HU_RemoteDistanceSet_L : simulink/Logic and Bit Operations/Bitwise Operator  logicop=AND  UseBitMask=on  BitMask=60  BitMaskRealWorld=Stored Integer
  HU_RemoteDistanceSet_O : Constant  Value=0  OutDataTypeStr=single
  HU_RemoteDistanceSet_S : ArithShift  BitShiftNumber=2
  HU_RemoteDistanceSet_Sub : Subsystem
  HU_RemoteDistanceSet_sat : Saturate  UpperLimit=15  LowerLimit=0
  HU_RemoteDistanceSetcv : DataTypeConversion
  HU_SEWEnable_Ad : Sum
  HU_SEWEnable_Convert : DataTypeConversion  OutDataTypeStr=uint32
  HU_SEWEnable_F : Gain
  HU_SEWEnable_L : simulink/Logic and Bit Operations/Bitwise Operator  logicop=AND  UseBitMask=on  BitMask=3  BitMaskRealWorld=Stored Integer
  HU_SEWEnable_O : Constant  Value=0  OutDataTypeStr=single
  HU_SEWEnable_S : ArithShift
  HU_SEWEnable_Sub : Subsystem
  HU_SEWEnable_sat : Saturate  UpperLimit=3  LowerLimit=0
  HU_SEWEnablecv : DataTypeConversion
  HU_SLASwitch_Ad : Sum
  HU_SLASwitch_Convert : DataTypeConversion  OutDataTypeStr=uint32
  HU_SLASwitch_F : Gain
  HU_SLASwitch_L : simulink/Logic and Bit Operations/Bitwise Operator  logicop=AND  UseBitMask=on  BitMask=8  BitMaskRealWorld=Stored Integer
  HU_SLASwitch_O : Constant  Value=0  OutDataTypeStr=single
  HU_SLASwitch_S : ArithShift  BitShiftNumber=3
  HU_SLASwitch_Sub : Subsystem
  HU_SLASwitch_sat : Saturate  UpperLimit=1  LowerLimit=0
  HU_SLASwitchcv : DataTypeConversion
  HU_Uls_BSD_Activation_Ad : Sum
  HU_Uls_BSD_Activation_Convert : DataTypeConversion  OutDataTypeStr=uint32
  HU_Uls_BSD_Activation_F : Gain
  HU_Uls_BSD_Activation_L : simulink/Logic and Bit Operations/Bitwise Operator  logicop=AND  UseBitMask=on  BitMask=3  BitMaskRealWorld=Stored Integer
  HU_Uls_BSD_Activation_O : Constant  Value=0  OutDataTypeStr=single
  HU_Uls_BSD_Activation_S : ArithShift
  HU_Uls_BSD_Activation_Sub : Subsystem
  HU_Uls_BSD_Activation_sat : Saturate  UpperLimit=3  LowerLimit=0
  HU_Uls_BSD_Activationcv : DataTypeConversion
  HU_Uls_FKP_Activation_Ad : Sum
  HU_Uls_FKP_Activation_Convert : DataTypeConversion  OutDataTypeStr=uint32
  HU_Uls_FKP_Activation_F : Gain
  HU_Uls_FKP_Activation_L : simulink/Logic and Bit Operations/Bitwise Operator  logicop=AND  UseBitMask=on  BitMask=48  BitMaskRealWorld=Stored Integer
  HU_Uls_FKP_Activation_O : Constant  Value=0  OutDataTypeStr=single
  HU_Uls_FKP_Activation_S : ArithShift  BitShiftNumber=4
  HU_Uls_FKP_Activation_Sub : Subsystem
  HU_Uls_FKP_Activation_sat : Saturate  UpperLimit=3  LowerLimit=0
  HU_Uls_FKP_Activationcv : DataTypeConversion
  HU_CTAEnable_Out : Outport
  HU_BSD_LCAEnable_Out : Outport  Port=2
  HU_LASModeSelection_Out : Outport  Port=3
  HU_LdwSensitivity_Out : Outport  Port=4
  HU_LASWarningModeSelection_Out : Outport  Port=5
  HU_SLASwitch_Out : Outport  Port=6
  HU_HMAEnable_Out : Outport  Port=7
  HU_RCWEnable_Out : Outport  Port=8
  HU_SEWEnable_Out : Outport  Port=9
  HU_RCWSoundEnable_Out : Outport  Port=10
  HU_LDWShakeLev_Out : Outport  Port=11
  HU_AudioWarningEnable_Out : Outport  Port=12
  HU_LockCtrlEnable_Out : Outport  Port=13
  HU_IACCEnable_Out : Outport  Port=14
  HU_OverspeedSoundWarEnable_Out : Outport  Port=15
  HU_OverspeedWarningEnable_Out : Outport  Port=16
  HU_OverspeedWarningOffset_Out : Outport  Port=17
  HU_Uls_BSD_Activation_Out : Outport  Port=18
  HU_LCATTCSetting_Out : Outport  Port=19
  HU_Uls_FKP_Activation_Out : Outport  Port=20
  HU_ParkingResume_Out : Outport  Port=21
  HU_DSMMemoryPositionFeedback_Out : Outport  Port=22
  HU_RemoteDistanceSet_Out : Outport  Port=23
  HU_ParkingConfirm_Out : Outport  Port=24
  HU_ObstacleSafeDistanceSet_Out : Outport  Port=25
  HU_DVRBrowseCommand_Out : Outport  Port=26
  wires:
  input/1 -> Demux/1
  HU_DVRBrowseCommandcv/1 -> HU_DVRBrowseCommand_F/1
  HU_DVRBrowseCommand_S/1 -> HU_DVRBrowseCommandcv/1
  HU_DVRBrowseCommand_L/1 -> HU_DVRBrowseCommand_S/1
  HU_DVRBrowseCommand_Convert/1 -> HU_DVRBrowseCommand_L/1
  HU_DVRBrowseCommand_Sub/1(Out1) -> HU_DVRBrowseCommand_Convert/1
  HU_DVRBrowseCommand_sat/1 -> HU_DVRBrowseCommand_Out/1
  HU_DVRBrowseCommand_Ad/1 -> HU_DVRBrowseCommand_sat/1
  HU_DVRBrowseCommand_O/1 -> HU_DVRBrowseCommand_Ad/2
  HU_DVRBrowseCommand_F/1 -> HU_DVRBrowseCommand_Ad/1
  HU_ObstacleSafeDistanceSetcv/1 -> HU_ObstacleSafeDistanceSet_F/1
  HU_ObstacleSafeDistanceSet_S/1 -> HU_ObstacleSafeDistanceSetcv/1
  HU_ObstacleSafeDistanceSet_L/1 -> HU_ObstacleSafeDistanceSet_S/1
  HU_ObstacleSafeDistanceSet_Convert/1 -> HU_ObstacleSafeDistanceSet_L/1
  HU_ObstacleSafeDistanceSet_Sub/1(Out1) -> HU_ObstacleSafeDistanceSet_Convert/1
  Demux/8 -> HU_DVRBrowseCommand_Sub/1(In1), HU_ObstacleSafeDistanceSet_Sub/1(In1)
  HU_ObstacleSafeDistanceSet_sat/1 -> HU_ObstacleSafeDistanceSet_Out/1
  HU_ObstacleSafeDistanceSet_Ad/1 -> HU_ObstacleSafeDistanceSet_sat/1
  HU_ObstacleSafeDistanceSet_O/1 -> HU_ObstacleSafeDistanceSet_Ad/2
  HU_ObstacleSafeDistanceSet_F/1 -> HU_ObstacleSafeDistanceSet_Ad/1
  HU_ParkingConfirmcv/1 -> HU_ParkingConfirm_F/1
  HU_ParkingConfirm_S/1 -> HU_ParkingConfirmcv/1
  HU_ParkingConfirm_L/1 -> HU_ParkingConfirm_S/1
  HU_ParkingConfirm_Convert/1 -> HU_ParkingConfirm_L/1
  HU_ParkingConfirm_Sub/1(Out1) -> HU_ParkingConfirm_Convert/1
  HU_ParkingConfirm_sat/1 -> HU_ParkingConfirm_Out/1
  HU_ParkingConfirm_Ad/1 -> HU_ParkingConfirm_sat/1
  HU_ParkingConfirm_O/1 -> HU_ParkingConfirm_Ad/2
  HU_ParkingConfirm_F/1 -> HU_ParkingConfirm_Ad/1
  HU_RemoteDistanceSetcv/1 -> HU_RemoteDistanceSet_F/1
  HU_RemoteDistanceSet_S/1 -> HU_RemoteDistanceSetcv/1
  HU_RemoteDistanceSet_L/1 -> HU_RemoteDistanceSet_S/1
  HU_RemoteDistanceSet_Convert/1 -> HU_RemoteDistanceSet_L/1
  HU_RemoteDistanceSet_Sub/1(Out1) -> HU_RemoteDistanceSet_Convert/1
  HU_RemoteDistanceSet_sat/1 -> HU_RemoteDistanceSet_Out/1
  HU_RemoteDistanceSet_Ad/1 -> HU_RemoteDistanceSet_sat/1
  HU_RemoteDistanceSet_O/1 -> HU_RemoteDistanceSet_Ad/2
  HU_RemoteDistanceSet_F/1 -> HU_RemoteDistanceSet_Ad/1
  HU_DSMMemoryPositionFeedbackcv/1 -> HU_DSMMemoryPositionFeedback_F/1
  HU_DSMMemoryPositionFeedback_S/1 -> HU_DSMMemoryPositionFeedbackcv/1
  HU_DSMMemoryPositionFeedback_L/1 -> HU_DSMMemoryPositionFeedback_S/1
  HU_DSMMemoryPositionFeedback_Convert/1 -> HU_DSMMemoryPositionFeedback_L/1
  HU_DSMMemoryPositionFeedback_Sub/1(Out1) -> HU_DSMMemoryPositionFeedback_Convert/1
  Demux/7 -> HU_ParkingConfirm_Sub/1(In1), HU_RemoteDistanceSet_Sub/1(In1), HU_DSMMemoryPositionFeedback_Sub/1(In1)
  HU_DSMMemoryPositionFeedback_sat/1 -> HU_DSMMemoryPositionFeedback_Out/1
  HU_DSMMemoryPositionFeedback_Ad/1 -> HU_DSMMemoryPositionFeedback_sat/1
  HU_DSMMemoryPositionFeedback_O/1 -> HU_DSMMemoryPositionFeedback_Ad/2
  HU_DSMMemoryPositionFeedback_F/1 -> HU_DSMMemoryPositionFeedback_Ad/1
  HU_ParkingResumecv/1 -> HU_ParkingResume_F/1
  HU_ParkingResume_S/1 -> HU_ParkingResumecv/1
  HU_ParkingResume_L/1 -> HU_ParkingResume_S/1
  HU_ParkingResume_Convert/1 -> HU_ParkingResume_L/1
  HU_ParkingResume_Sub/1(Out1) -> HU_ParkingResume_Convert/1
  HU_ParkingResume_sat/1 -> HU_ParkingResume_Out/1
  HU_ParkingResume_Ad/1 -> HU_ParkingResume_sat/1
  HU_ParkingResume_O/1 -> HU_ParkingResume_Ad/2
  HU_ParkingResume_F/1 -> HU_ParkingResume_Ad/1
  HU_Uls_FKP_Activationcv/1 -> HU_Uls_FKP_Activation_F/1
  HU_Uls_FKP_Activation_S/1 -> HU_Uls_FKP_Activationcv/1
  HU_Uls_FKP_Activation_L/1 -> HU_Uls_FKP_Activation_S/1
  HU_Uls_FKP_Activation_Convert/1 -> HU_Uls_FKP_Activation_L/1
  HU_Uls_FKP_Activation_Sub/1(Out1) -> HU_Uls_FKP_Activation_Convert/1
  HU_Uls_FKP_Activation_sat/1 -> HU_Uls_FKP_Activation_Out/1
  HU_Uls_FKP_Activation_Ad/1 -> HU_Uls_FKP_Activation_sat/1
  HU_Uls_FKP_Activation_O/1 -> HU_Uls_FKP_Activation_Ad/2
  HU_Uls_FKP_Activation_F/1 -> HU_Uls_FKP_Activation_Ad/1
  HU_LCATTCSettingcv/1 -> HU_LCATTCSetting_F/1
  HU_LCATTCSetting_S/1 -> HU_LCATTCSettingcv/1
  HU_LCATTCSetting_L/1 -> HU_LCATTCSetting_S/1
  HU_LCATTCSetting_Convert/1 -> HU_LCATTCSetting_L/1
  HU_LCATTCSetting_Sub/1(Out1) -> HU_LCATTCSetting_Convert/1
  HU_LCATTCSetting_sat/1 -> HU_LCATTCSetting_Out/1
  HU_LCATTCSetting_Ad/1 -> HU_LCATTCSetting_sat/1
  HU_LCATTCSetting_O/1 -> HU_LCATTCSetting_Ad/2
  HU_LCATTCSetting_F/1 -> HU_LCATTCSetting_Ad/1
  HU_Uls_BSD_Activationcv/1 -> HU_Uls_BSD_Activation_F/1
  HU_Uls_BSD_Activation_S/1 -> HU_Uls_BSD_Activationcv/1
  HU_Uls_BSD_Activation_L/1 -> HU_Uls_BSD_Activation_S/1
  HU_Uls_BSD_Activation_Convert/1 -> HU_Uls_BSD_Activation_L/1
  HU_Uls_BSD_Activation_Sub/1(Out1) -> HU_Uls_BSD_Activation_Convert/1
  Demux/6 -> HU_ParkingResume_Sub/1(In1), HU_Uls_FKP_Activation_Sub/1(In1), HU_LCATTCSetting_Sub/1(In1), HU_Uls_BSD_Activation_Sub/1(In1)
  HU_Uls_BSD_Activation_sat/1 -> HU_Uls_BSD_Activation_Out/1
  HU_Uls_BSD_Activation_Ad/1 -> HU_Uls_BSD_Activation_sat/1
  HU_Uls_BSD_Activation_O/1 -> HU_Uls_BSD_Activation_Ad/2
  HU_Uls_BSD_Activation_F/1 -> HU_Uls_BSD_Activation_Ad/1
  HU_OverspeedWarningOffsetcv/1 -> HU_OverspeedWarningOffset_F/1
  HU_OverspeedWarningOffset_S/1 -> HU_OverspeedWarningOffsetcv/1
  HU_OverspeedWarningOffset_L/1 -> HU_OverspeedWarningOffset_S/1
  HU_OverspeedWarningOffset_Convert/1 -> HU_OverspeedWarningOffset_L/1
  HU_OverspeedWarningOffset_Sub/1(Out1) -> HU_OverspeedWarningOffset_Convert/1
  HU_OverspeedWarningOffset_sat/1 -> HU_OverspeedWarningOffset_Out/1
  HU_OverspeedWarningOffset_Ad/1 -> HU_OverspeedWarningOffset_sat/1
  HU_OverspeedWarningOffset_O/1 -> HU_OverspeedWarningOffset_Ad/2
  HU_OverspeedWarningOffset_F/1 -> HU_OverspeedWarningOffset_Ad/1
  HU_OverspeedWarningEnablecv/1 -> HU_OverspeedWarningEnable_F/1
  HU_OverspeedWarningEnable_S/1 -> HU_OverspeedWarningEnablecv/1
  HU_OverspeedWarningEnable_L/1 -> HU_OverspeedWarningEnable_S/1
  HU_OverspeedWarningEnable_Convert/1 -> HU_OverspeedWarningEnable_L/1
  HU_OverspeedWarningEnable_Sub/1(Out1) -> HU_OverspeedWarningEnable_Convert/1
  Demux/5 -> HU_OverspeedWarningOffset_Sub/1(In1), HU_OverspeedWarningEnable_Sub/1(In1)
  HU_OverspeedWarningEnable_sat/1 -> HU_OverspeedWarningEnable_Out/1
  HU_OverspeedWarningEnable_Ad/1 -> HU_OverspeedWarningEnable_sat/1
  HU_OverspeedWarningEnable_O/1 -> HU_OverspeedWarningEnable_Ad/2
  HU_OverspeedWarningEnable_F/1 -> HU_OverspeedWarningEnable_Ad/1
  HU_OverspeedSoundWarEnablecv/1 -> HU_OverspeedSoundWarEnable_F/1
  HU_OverspeedSoundWarEnable_S/1 -> HU_OverspeedSoundWarEnablecv/1
  HU_OverspeedSoundWarEnable_L/1 -> HU_OverspeedSoundWarEnable_S/1
  HU_OverspeedSoundWarEnable_Convert/1 -> HU_OverspeedSoundWarEnable_L/1
  HU_OverspeedSoundWarEnable_Sub/1(Out1) -> HU_OverspeedSoundWarEnable_Convert/1
  HU_OverspeedSoundWarEnable_sat/1 -> HU_OverspeedSoundWarEnable_Out/1
  HU_OverspeedSoundWarEnable_Ad/1 -> HU_OverspeedSoundWarEnable_sat/1
  HU_OverspeedSoundWarEnable_O/1 -> HU_OverspeedSoundWarEnable_Ad/2
  HU_OverspeedSoundWarEnable_F/1 -> HU_OverspeedSoundWarEnable_Ad/1
  HU_IACCEnablecv/1 -> HU_IACCEnable_F/1
  HU_IACCEnable_S/1 -> HU_IACCEnablecv/1
  HU_IACCEnable_L/1 -> HU_IACCEnable_S/1
  HU_IACCEnable_Convert/1 -> HU_IACCEnable_L/1
  HU_IACCEnable_Sub/1(Out1) -> HU_IACCEnable_Convert/1
  HU_IACCEnable_sat/1 -> HU_IACCEnable_Out/1
  HU_IACCEnable_Ad/1 -> HU_IACCEnable_sat/1
  HU_IACCEnable_O/1 -> HU_IACCEnable_Ad/2
  HU_IACCEnable_F/1 -> HU_IACCEnable_Ad/1
  HU_LockCtrlEnablecv/1 -> HU_LockCtrlEnable_F/1
  HU_LockCtrlEnable_S/1 -> HU_LockCtrlEnablecv/1
  HU_LockCtrlEnable_L/1 -> HU_LockCtrlEnable_S/1
  HU_LockCtrlEnable_Convert/1 -> HU_LockCtrlEnable_L/1
  HU_LockCtrlEnable_Sub/1(Out1) -> HU_LockCtrlEnable_Convert/1
  HU_LockCtrlEnable_sat/1 -> HU_LockCtrlEnable_Out/1
  HU_LockCtrlEnable_Ad/1 -> HU_LockCtrlEnable_sat/1
  HU_LockCtrlEnable_O/1 -> HU_LockCtrlEnable_Ad/2
  HU_LockCtrlEnable_F/1 -> HU_LockCtrlEnable_Ad/1
  HU_AudioWarningEnablecv/1 -> HU_AudioWarningEnable_F/1
  HU_AudioWarningEnable_S/1 -> HU_AudioWarningEnablecv/1
  HU_AudioWarningEnable_L/1 -> HU_AudioWarningEnable_S/1
  HU_AudioWarningEnable_Convert/1 -> HU_AudioWarningEnable_L/1
  HU_AudioWarningEnable_Sub/1(Out1) -> HU_AudioWarningEnable_Convert/1
  Demux/4 -> HU_OverspeedSoundWarEnable_Sub/1(In1), HU_IACCEnable_Sub/1(In1), HU_LockCtrlEnable_Sub/1(In1), HU_AudioWarningEnable_Sub/1(In1)
  HU_AudioWarningEnable_sat/1 -> HU_AudioWarningEnable_Out/1
  HU_AudioWarningEnable_Ad/1 -> HU_AudioWarningEnable_sat/1
  HU_AudioWarningEnable_O/1 -> HU_AudioWarningEnable_Ad/2
  HU_AudioWarningEnable_F/1 -> HU_AudioWarningEnable_Ad/1
  HU_LDWShakeLevcv/1 -> HU_LDWShakeLev_F/1
  HU_LDWShakeLev_S/1 -> HU_LDWShakeLevcv/1
  HU_LDWShakeLev_L/1 -> HU_LDWShakeLev_S/1
  HU_LDWShakeLev_Convert/1 -> HU_LDWShakeLev_L/1
  HU_LDWShakeLev_Sub/1(Out1) -> HU_LDWShakeLev_Convert/1
  HU_LDWShakeLev_sat/1 -> HU_LDWShakeLev_Out/1
  HU_LDWShakeLev_Ad/1 -> HU_LDWShakeLev_sat/1
  HU_LDWShakeLev_O/1 -> HU_LDWShakeLev_Ad/2
  HU_LDWShakeLev_F/1 -> HU_LDWShakeLev_Ad/1
  HU_RCWSoundEnablecv/1 -> HU_RCWSoundEnable_F/1
  HU_RCWSoundEnable_S/1 -> HU_RCWSoundEnablecv/1
  HU_RCWSoundEnable_L/1 -> HU_RCWSoundEnable_S/1
  HU_RCWSoundEnable_Convert/1 -> HU_RCWSoundEnable_L/1
  HU_RCWSoundEnable_Sub/1(Out1) -> HU_RCWSoundEnable_Convert/1
  HU_RCWSoundEnable_sat/1 -> HU_RCWSoundEnable_Out/1
  HU_RCWSoundEnable_Ad/1 -> HU_RCWSoundEnable_sat/1
  HU_RCWSoundEnable_O/1 -> HU_RCWSoundEnable_Ad/2
  HU_RCWSoundEnable_F/1 -> HU_RCWSoundEnable_Ad/1
  HU_SEWEnablecv/1 -> HU_SEWEnable_F/1
  HU_SEWEnable_S/1 -> HU_SEWEnablecv/1
  HU_SEWEnable_L/1 -> HU_SEWEnable_S/1
  HU_SEWEnable_Convert/1 -> HU_SEWEnable_L/1
  HU_SEWEnable_Sub/1(Out1) -> HU_SEWEnable_Convert/1
  Demux/3 -> HU_LDWShakeLev_Sub/1(In1), HU_RCWSoundEnable_Sub/1(In1), HU_SEWEnable_Sub/1(In1)
  HU_SEWEnable_sat/1 -> HU_SEWEnable_Out/1
  HU_SEWEnable_Ad/1 -> HU_SEWEnable_sat/1
  HU_SEWEnable_O/1 -> HU_SEWEnable_Ad/2
  HU_SEWEnable_F/1 -> HU_SEWEnable_Ad/1
  HU_RCWEnablecv/1 -> HU_RCWEnable_F/1
  HU_RCWEnable_S/1 -> HU_RCWEnablecv/1
  HU_RCWEnable_L/1 -> HU_RCWEnable_S/1
  HU_RCWEnable_Convert/1 -> HU_RCWEnable_L/1
  HU_RCWEnable_Sub/1(Out1) -> HU_RCWEnable_Convert/1
  HU_RCWEnable_sat/1 -> HU_RCWEnable_Out/1
  HU_RCWEnable_Ad/1 -> HU_RCWEnable_sat/1
  HU_RCWEnable_O/1 -> HU_RCWEnable_Ad/2
  HU_RCWEnable_F/1 -> HU_RCWEnable_Ad/1
  HU_HMAEnablecv/1 -> HU_HMAEnable_F/1
  HU_HMAEnable_S/1 -> HU_HMAEnablecv/1
  HU_HMAEnable_L/1 -> HU_HMAEnable_S/1
  HU_HMAEnable_Convert/1 -> HU_HMAEnable_L/1
  HU_HMAEnable_Sub/1(Out1) -> HU_HMAEnable_Convert/1
  HU_HMAEnable_sat/1 -> HU_HMAEnable_Out/1
  HU_HMAEnable_Ad/1 -> HU_HMAEnable_sat/1
  HU_HMAEnable_O/1 -> HU_HMAEnable_Ad/2
  HU_HMAEnable_F/1 -> HU_HMAEnable_Ad/1
  HU_SLASwitchcv/1 -> HU_SLASwitch_F/1
  HU_SLASwitch_S/1 -> HU_SLASwitchcv/1
  HU_SLASwitch_L/1 -> HU_SLASwitch_S/1
  HU_SLASwitch_Convert/1 -> HU_SLASwitch_L/1
  HU_SLASwitch_Sub/1(Out1) -> HU_SLASwitch_Convert/1
  HU_SLASwitch_sat/1 -> HU_SLASwitch_Out/1
  HU_SLASwitch_Ad/1 -> HU_SLASwitch_sat/1
  HU_SLASwitch_O/1 -> HU_SLASwitch_Ad/2
  HU_SLASwitch_F/1 -> HU_SLASwitch_Ad/1
  HU_LASWarningModeSelectioncv/1 -> HU_LASWarningModeSelection_F/1
  HU_LASWarningModeSelection_S/1 -> HU_LASWarningModeSelectioncv/1
  HU_LASWarningModeSelection_L/1 -> HU_LASWarningModeSelection_S/1
  HU_LASWarningModeSelection_Convert/1 -> HU_LASWarningModeSelection_L/1
  HU_LASWarningModeSelection_Sub/1(Out1) -> HU_LASWarningModeSelection_Convert/1
  HU_LASWarningModeSelection_sat/1 -> HU_LASWarningModeSelection_Out/1
  HU_LASWarningModeSelection_Ad/1 -> HU_LASWarningModeSelection_sat/1
  HU_LASWarningModeSelection_O/1 -> HU_LASWarningModeSelection_Ad/2
  HU_LASWarningModeSelection_F/1 -> HU_LASWarningModeSelection_Ad/1
  HU_LdwSensitivitycv/1 -> HU_LdwSensitivity_F/1
  HU_LdwSensitivity_S/1 -> HU_LdwSensitivitycv/1
  HU_LdwSensitivity_L/1 -> HU_LdwSensitivity_S/1
  HU_LdwSensitivity_Convert/1 -> HU_LdwSensitivity_L/1
  HU_LdwSensitivity_Sub/1(Out1) -> HU_LdwSensitivity_Convert/1
  HU_LdwSensitivity_sat/1 -> HU_LdwSensitivity_Out/1
  HU_LdwSensitivity_Ad/1 -> HU_LdwSensitivity_sat/1
  HU_LdwSensitivity_O/1 -> HU_LdwSensitivity_Ad/2
  HU_LdwSensitivity_F/1 -> HU_LdwSensitivity_Ad/1
  HU_LASModeSelectioncv/1 -> HU_LASModeSelection_F/1
  HU_LASModeSelection_S/1 -> HU_LASModeSelectioncv/1
  HU_LASModeSelection_L/1 -> HU_LASModeSelection_S/1
  HU_LASModeSelection_Convert/1 -> HU_LASModeSelection_L/1
  HU_LASModeSelection_Sub/1(Out1) -> HU_LASModeSelection_Convert/1
  HU_LASModeSelection_sat/1 -> HU_LASModeSelection_Out/1
  HU_LASModeSelection_Ad/1 -> HU_LASModeSelection_sat/1
  HU_LASModeSelection_O/1 -> HU_LASModeSelection_Ad/2
  HU_LASModeSelection_F/1 -> HU_LASModeSelection_Ad/1
  HU_BSD_LCAEnablecv/1 -> HU_BSD_LCAEnable_F/1
  HU_BSD_LCAEnable_S/1 -> HU_BSD_LCAEnablecv/1
  HU_BSD_LCAEnable_L/1 -> HU_BSD_LCAEnable_S/1
  HU_BSD_LCAEnable_Convert/1 -> HU_BSD_LCAEnable_L/1
  HU_BSD_LCAEnable_Sub/1(Out1) -> HU_BSD_LCAEnable_Convert/1
  HU_BSD_LCAEnable_sat/1 -> HU_BSD_LCAEnable_Out/1
  HU_BSD_LCAEnable_Ad/1 -> HU_BSD_LCAEnable_sat/1
  HU_BSD_LCAEnable_O/1 -> HU_BSD_LCAEnable_Ad/2
  HU_BSD_LCAEnable_F/1 -> HU_BSD_LCAEnable_Ad/1
  HU_CTAEnablecv/1 -> HU_CTAEnable_F/1
  HU_CTAEnable_S/1 -> HU_CTAEnablecv/1
  HU_CTAEnable_L/1 -> HU_CTAEnable_S/1
  HU_CTAEnable_Convert/1 -> HU_CTAEnable_L/1
  HU_CTAEnable_Sub/1(Out1) -> HU_CTAEnable_Convert/1
  HU_CTAEnableinput1_Ad/1 -> HU_CTAEnable_Sub/1(In1)
  Demux/2 -> HU_RCWEnable_Sub/1(In1), HU_HMAEnable_Sub/1(In1), HU_SLASwitch_Sub/1(In1), HU_LASWarningModeSelection_Sub/1(In1), HU_CTAEnableinput1_Ad/2
  HU_CTAEnableinput1_P/1 -> HU_CTAEnableinput1_Ad/1
  HU_CTAEnableinput1_C/1 -> HU_CTAEnableinput1_P/2
  Demux/1 -> HU_LdwSensitivity_Sub/1(In1), HU_LASModeSelection_Sub/1(In1), HU_BSD_LCAEnable_Sub/1(In1), HU_CTAEnableinput1_P/1
  HU_CTAEnable_sat/1 -> HU_CTAEnable_Out/1
  HU_CTAEnable_Ad/1 -> HU_CTAEnable_sat/1
  HU_CTAEnable_O/1 -> HU_CTAEnable_Ad/2
  HU_CTAEnable_F/1 -> HU_CTAEnable_Ad/1
